simulink model "excercise1_2bd"  (R2023b)
settings: Solver=VariableStepAuto  StartTime=0.0  StopTime=10.0  RelTol=1e-3
undefined symbols (not defined in the file): d, k, m
settings Model: Creator=elliot  LastModifiedBy=elliot

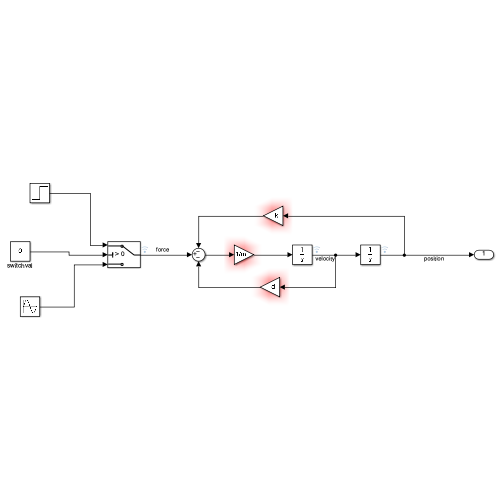
[thumbnail: Simulink's stored preview of the top-level diagram]
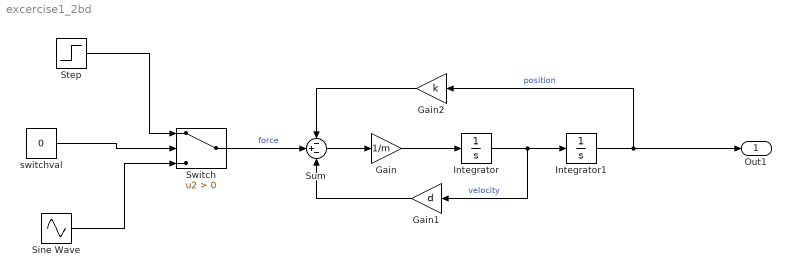
== system excercise1_2bd ==
  Gain : Gain  Gain=1/m
  Gain1 : Gain  Gain=d
  Gain2 : Gain  Gain=k
  Integrator : Integrator
  Integrator1 : Integrator
  Sine Wave : Sin  Frequency=10  SampleTime=0
  Step : Step  Time=0  SampleTime=0
  Sum : Sum  Inputs=-+-
  Switch : Switch  Criteria=u2 > Threshold  SaturateOnIntegerOverflow=off  InputSameDT=off
  switchval : Constant  Value=0
  Out1 : Outport
  wires:
  Gain/1 -> Integrator/1
  Sum/1 -> Gain/1
  switchval/1 -> Switch/2
  Sine Wave/1 -> Switch/3
  Gain1/1 -> Sum/3
  Switch/1 -> Sum/2  "force"
  Step/1 -> Switch/1
  Integrator/1 -> Integrator1/1, Gain1/1  "velocity"
  Integrator1/1 -> Gain2/1, Out1/1  "position"
  Gain2/1 -> Sum/1
